simulink model "wmr_cmd_vel_publisher"  (R2018b)
settings: Solver=VariableStepAuto  StartTime=0.0  StopTime=10  RelTol=1e-3
undefined symbols (not defined in the file or in its folder): Angular, Linear
libraries: robotlib x2
settings Model: Creator=robot  LastModifiedBy=robot

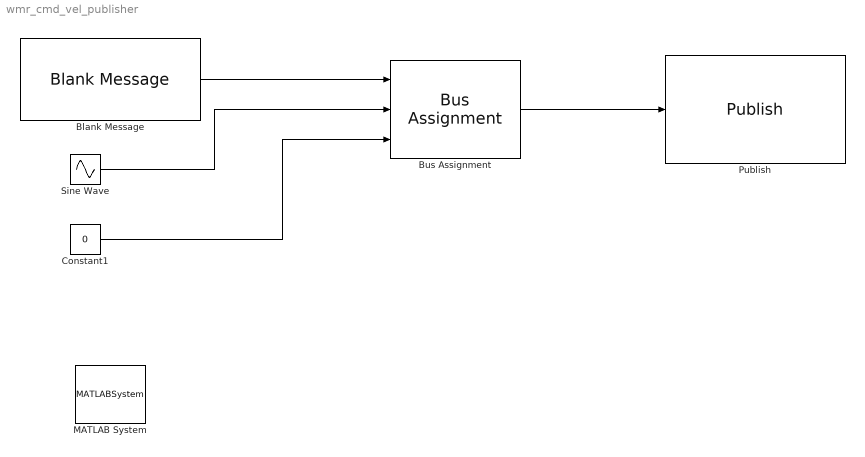
== system wmr_cmd_vel_publisher ==
  Blank Message : robotlib/Blank Message  messageClass=Message  entityType=geometry_msgs/Twist  messageType=geometry_msgs/Twist  SampleTime=inf
      settings: SourceProductBaseCode=RO
  Bus Assignment : BusAssignment  AssignedSignals=Linear.X,Angular.Z
  Constant1 : Constant  Value=0
  MATLAB System : MATLABSystem  System=ros_rate  RATE=[0.5]  SimulateUsing=Code generation
      mask Type: ros_rate
      mask Display: disp('ros_rate');
  Publish : robotlib/Publish  topicSource=Select from ROS network  topic=/cmd_vel  messageType=geometry_msgs/Twist  messageQueueLength=1
      settings: SourceProductBaseCode=RO
  Sine Wave : Sin  Frequency=10  SampleTime=0
  wires:
  Bus Assignment/1 -> Publish/1
  Blank Message/1 -> Bus Assignment/1
  Sine Wave/1 -> Bus Assignment/2
  Constant1/1 -> Bus Assignment/3
